simulink model "viteza_reactie"  (R2021a)
settings: Solver=VariableStepAuto  StartTime=0.0  StopTime=10.0  RelTol=1e-3
values from neighbouring files (symbols this model uses):
  EdR = 49584/8.32    (= 5959.61538462)    [script.m]
  k0 = 34930800    [script.m]
settings Model: Creator=Automatica  LastModifiedBy=Automatica

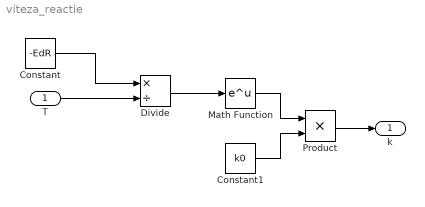
== system viteza_reactie ==
  T : Inport
  Constant : Constant  Value=-EdR
  Constant1 : Constant  Value=k0
  Divide : Product  Inputs=*/
  Math Function : Math  SaturateOnIntegerOverflow=on
  Product : Product
  k : Outport
  wires:
  T/1 -> Divide/2
  Constant/1 -> Divide/1
  Divide/1 -> Math Function/1
  Math Function/1 -> Product/1
  Constant1/1 -> Product/2
  Product/1 -> k/1
